simulink model "cdma_anti_jamming_system"  (R2020b)
settings: Solver=VariableStepAuto  StartTime=0.0  StopTime=0.004  RelTol=1e-3
undefined symbols (not defined in the file): fdesignblkfcn, gcbh
libraries: commutil2 x5, commfilt2 x1, commchan3 x1, commrandsrc3 x1, commseqgen3 x1
settings Model: Creator=joycelai  LastModifiedBy=joycelai

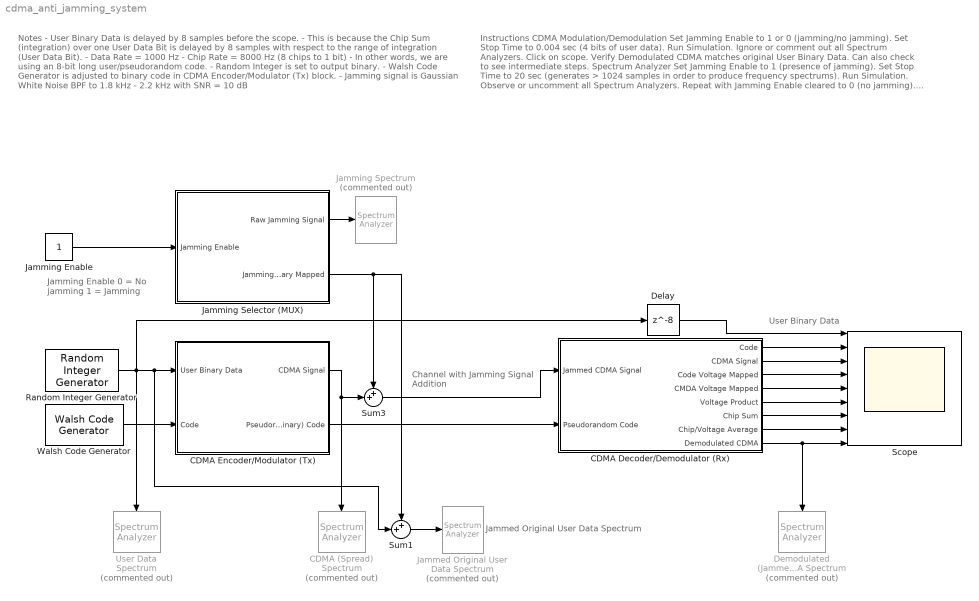
== system cdma_anti_jamming_system ==
  note: Jammed Original User Data Spectrum
  note: Jamming Enable
      | 0 = No jamming
      | 1 = Jamming
  note: Notes
      |
      | - User Binary Data is delayed by 8 samples before the scope.
      | - This is because the Chip Sum (integration) over one User Data Bit is delayed by 8 samples with respect to the range of integration (User Data Bit).
      |
      | - Data Rate = 1000 Hz
      | - Chip Rate = 8000 Hz (8 chips to 1 bit)
      | - In other words, we are using an 8-bit long user/pseudorandom code.
      | - Random Integer is set to output binary.
      | - Walsh Code Generator is adjusted to binary code in CDMA Encoder/Modulator (Tx) block.
      | - Jamming signal is Gaussian White Noise BPF to 1.8 kHz - 2.2 kHz with SNR = 10 dB
  note: Instructions
      |
      | CDMA Modulation/Demodulation
      |
      | Set Jamming Enable to 1 or 0 (jamming/no jamming).
      | Set Stop Time to 0.004 sec (4 bits of user data).
      | Run Simulation.
      | Ignore or comment out all Spectrum Analyzers.
      | Click on scope.
      | Verify Demodulated CDMA matches original User Binary Data.
      | Can also check to see intermediate steps.
      |
      | Spectrum Analyzer
      |
      | Set Jamming Enable to 1 (presence of jamming).
      | Set Stop Time to 20 sec (generates > 1024 samples in order to produce frequency spectrums).
      | Run Simulation.
      | Observe or uncomment all Spectrum Analyzers.
      | Repeat with Jamming Enable cleared to 0 (no jamming).
      | Verify that the Demodulated (Jammed) CDMA Spectrum mirrors the User Data Spectrum.
  note: User Binary Data
  note: Channel with Jamming Signal Addition
  CDMA (Spread) Spectrum : SpectrumAnalyzer  Commented=on
  CDMA Decoder/Demodulator (Rx) : Subsystem
  CDMA Encoder/Modulator (Tx) : Subsystem
  Delay : Delay  DelayLength=8  InitialCondition=0  SampleTime=1/(1000*8)
  Demodulated (Jammed) CDMA Spectrum : SpectrumAnalyzer  Commented=on
  Jammed Original User Data Spectrum : SpectrumAnalyzer  Commented=on
  Jamming Enable : Constant
  Jamming Selector (MUX) : Subsystem
  Jamming Spectrum : SpectrumAnalyzer  Commented=on
  Random Integer Generator : commrandsrc3/Random Integer Generator  SetSize=2  SeedSource=Auto  Seed=10  SampleTime=1/1000  SamplesPerFrame=1  OutputDataType=double  SimulateUsing=Interpreted execution
  Scope : Scope  NumInputPorts=9
  Sum1 : Sum  Inputs=++|
  Sum3 : Sum  Inputs=++|
  User Data Spectrum : SpectrumAnalyzer  Commented=on
  Walsh Code Generator : commseqgen3/Walsh Code Generator  Length=8  Index=5  SampleTime=1/(1000*8)  SamplesPerFrame=1  OutputDataType=double  SimulateUsing=Code generation
      settings: SourceProductBaseCode=CM
  wires:
  Walsh Code Generator/1 -> CDMA Encoder/Modulator (Tx)/2(Code)
  Sum3/1 -> CDMA Decoder/Demodulator (Rx)/1(Jammed CDMA Signal)
  CDMA Decoder/Demodulator (Rx)/8(Demodulated CDMA) -> Scope/9, Demodulated (Jammed) CDMA Spectrum/1
  Random Integer Generator/1 -> CDMA Encoder/Modulator (Tx)/1(User Binary Data), Sum1/2, Delay/1, User Data Spectrum/1
  Jamming Selector (MUX)/1(Raw Jamming Signal) -> Jamming Spectrum/1
  Jamming Selector (MUX)/2(Jamming Binary Mapped) -> Sum3/1, Sum1/1
  Jamming Enable/1 -> Jamming Selector (MUX)/1(Jamming Enable)
  CDMA Decoder/Demodulator (Rx)/7(Chip/Voltage Average) -> Scope/8
  CDMA Decoder/Demodulator (Rx)/6(Chip Sum) -> Scope/7
  CDMA Decoder/Demodulator (Rx)/5(Voltage Product) -> Scope/6
  CDMA Decoder/Demodulator (Rx)/4(CMDA Voltage Mapped) -> Scope/5
  CDMA Decoder/Demodulator (Rx)/3(Code Voltage Mapped) -> Scope/4
  CDMA Decoder/Demodulator (Rx)/2(CDMA Signal) -> Scope/3
  CDMA Decoder/Demodulator (Rx)/1(Code) -> Scope/2
  CDMA Encoder/Modulator (Tx)/2(Pseudorandom (Binary) Code) -> CDMA Decoder/Demodulator (Rx)/2(Pseudorandom Code)
  Delay/1 -> Scope/1
  Sum1/1 -> Jammed Original User Data Spectrum/1
  CDMA Encoder/Modulator (Tx)/1(CDMA Signal) -> Sum3/2, CDMA (Spread) Spectrum/1

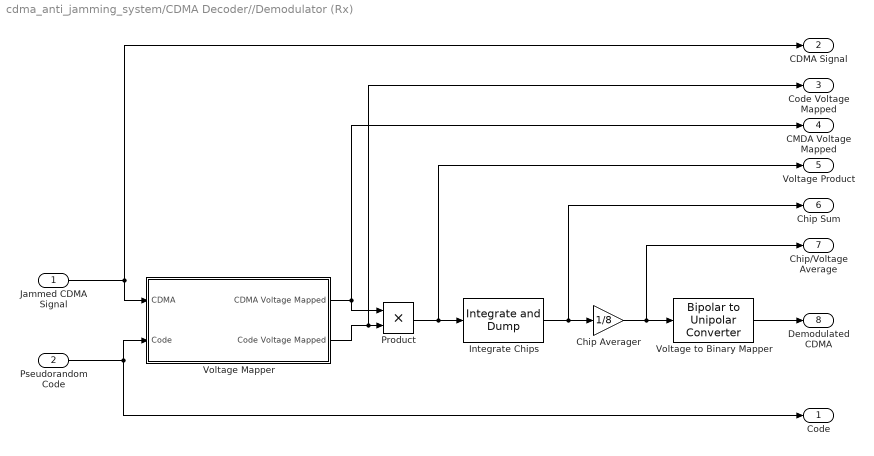
== system cdma_anti_jamming_system/CDMA Decoder//Demodulator (Rx) ==
  Jammed CDMA Signal : Inport
  Pseudorandom Code : Inport  Port=2
  Chip Averager : Gain  Gain=1/8
  Integrate Chips : commfilt2/Integrate and Dump  obssamples=8  offsetsamples=0  nodump=off  roundingMode=Floor  overflowMode=off  outputDataTypeStr=Inherit: Same as accumulator  outputLastDataTypeStr=Inherit: Same as accumulator
  Product : Product
  Voltage Mapper : Subsystem
  Voltage to Binary Mapper : commutil2/Bipolar to Unipolar Converter  M=2  polarity=Negative  dataType=Inherit via internal rule
      settings: SourceProductBaseCode=CM
  Code : Outport
  CDMA Signal : Outport  Port=2
  Code Voltage Mapped : Outport  Port=3
  CMDA Voltage Mapped : Outport  Port=4
  Voltage Product : Outport  Port=5
  Chip Sum : Outport  Port=6
  Chip/Voltage Average : Outport  Port=7
  Demodulated CDMA : Outport  Port=8
  wires:
  Chip Averager/1 -> Chip/Voltage Average/1, Voltage to Binary Mapper/1
  Voltage to Binary Mapper/1 -> Demodulated CDMA/1
  Voltage Mapper/2(Code Voltage Mapped) -> Code Voltage Mapped/1, Product/2
  Integrate Chips/1 -> Chip Sum/1, Chip Averager/1
  Voltage Mapper/1(CDMA Voltage Mapped) -> Product/1, CMDA Voltage Mapped/1
  Product/1 -> Voltage Product/1, Integrate Chips/1
  Jammed CDMA Signal/1 -> CDMA Signal/1, Voltage Mapper/1(CDMA)
  Pseudorandom Code/1 -> Code/1, Voltage Mapper/2(Code)

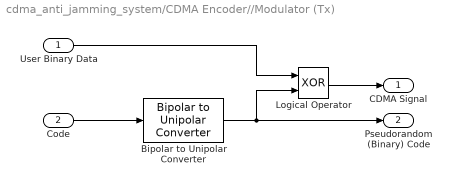
== system cdma_anti_jamming_system/CDMA Encoder//Modulator (Tx) ==
  User Binary Data : Inport
  Code : Inport  Port=2
  Bipolar to Unipolar Converter : commutil2/Bipolar to Unipolar Converter  M=2  polarity=Positive  dataType=Inherit via internal rule
      settings: SourceProductBaseCode=CM
  Logical Operator : Logic  Operator=XOR  AllPortsSameDT=off  OutDataTypeStr=boolean
  CDMA Signal : Outport
  Pseudorandom (Binary) Code : Outport  Port=2
  wires:
  User Binary Data/1 -> Logical Operator/1
  Code/1 -> Bipolar to Unipolar Converter/1
  Bipolar to Unipolar Converter/1 -> Pseudorandom (Binary) Code/1, Logical Operator/2
  Logical Operator/1 -> CDMA Signal/1

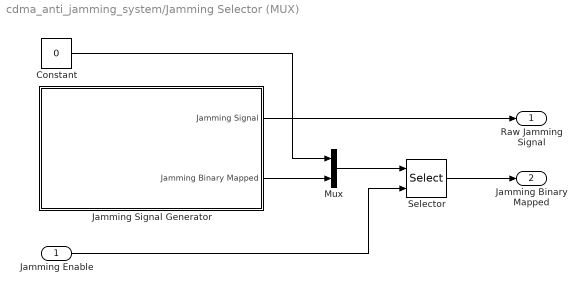
== system cdma_anti_jamming_system/Jamming Selector (MUX) ==
  Jamming Enable : Inport
  Constant : Constant  Value=0  SampleTime=1/1000
  Jamming Signal Generator : Subsystem
  Mux : Mux  Inputs=2
  Selector : Selector  IndexMode=Zero-based  InputPortWidth=2  IndexOptions=Index vector (port)  Indices=0  OutputSizes=1
  Raw Jamming Signal : Outport
  Jamming Binary Mapped : Outport  Port=2
  wires:
  Jamming Signal Generator/2(Jamming Binary Mapped) -> Mux/2
  Constant/1 -> Mux/1
  Selector/1 -> Jamming Binary Mapped/1
  Jamming Signal Generator/1(Jamming Signal) -> Raw Jamming Signal/1
  Mux/1 -> Selector/1
  Jamming Enable/1 -> Selector/2

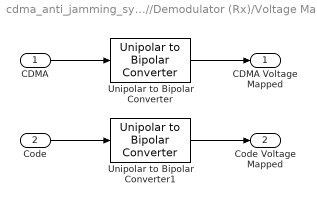
== system cdma_anti_jamming_system/CDMA Decoder//Demodulator (Rx)/Voltage Mapper ==
  CDMA : Inport
  Code : Inport  Port=2
  Unipolar to Bipolar Converter : commutil2/Unipolar to Bipolar Converter  M=2  polarity=Negative  dataType=Inherit via internal rule
  Unipolar to Bipolar Converter1 : commutil2/Unipolar to Bipolar Converter  M=2  polarity=Negative  dataType=Inherit via internal rule
  CDMA Voltage Mapped : Outport
  Code Voltage Mapped : Outport  Port=2
  wires:
  CDMA/1 -> Unipolar to Bipolar Converter/1
  Code/1 -> Unipolar to Bipolar Converter1/1
  Unipolar to Bipolar Converter/1 -> CDMA Voltage Mapped/1
  Unipolar to Bipolar Converter1/1 -> Code Voltage Mapped/1

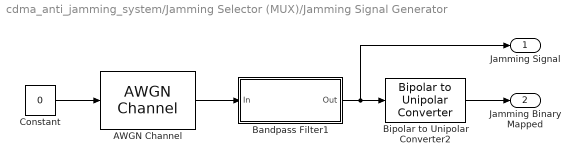
== system cdma_anti_jamming_system/Jamming Selector (MUX)/Jamming Signal Generator ==
  AWGN Channel : commchan3/AWGN Channel  InputProcessing=Columns as channels (frame based)  seed=67  noiseMode="Signal to noise ratio  (SNR)"  EbNodB=10  EsNodB=10  SNRdB=10  bitsPerSym=1  Ps=1  Tsym=1  variance=1
  Bandpass Filter1 : Subsystem  DialogController=fdesignblkfcn  InitFcn=fdesignblkfcn(gcbh, {'InitFcn'});  mask(Bandpass Filter){}
      mask help: Design a bandpass filter
      settings: CopyFcn=fdesignblkfcn(gcbh, {'CopyFcn'});
      mask Help: helpview(mapfilelocation('dsp'), 'dspbandpassfilter');
      mask Display: disp('Bandpass');
  Bipolar to Unipolar Converter2 : commutil2/Bipolar to Unipolar Converter  M=2  polarity=Positive  dataType=Inherit via internal rule
      settings: SourceProductBaseCode=CM
  Constant : Constant  Value=0  SampleTime=1/1000
  Jamming Signal : Outport
  Jamming Binary Mapped : Outport  Port=2
  wires:
  Constant/1 -> AWGN Channel/1
  AWGN Channel/1 -> Bandpass Filter1/1(In)
  Bipolar to Unipolar Converter2/1 -> Jamming Binary Mapped/1
  Bandpass Filter1/1(Out) -> Jamming Signal/1, Bipolar to Unipolar Converter2/1

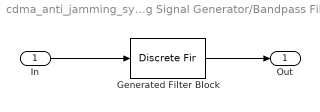
== system cdma_anti_jamming_system/Jamming Selector (MUX)/Jamming Signal Generator/Bandpass Filter1 ==
  In : Inport
  Generated Filter Block : DiscreteFir  Tag=BlockMethodSubSystem  Coefficients=[-0.0008992291487744296 0.0016414518747943749 0.0031352071842225397 -0.0040707550828814922 -0.0063731852227904111 0.0074874286806090491 0.0098354319566295711 -0.010189316513446216 -0.011302794465874122 0.0096929185841818435 0.0079428653987464216 -0.0031368247881221642 0.0028299878877943137 -0.011508674243001471 -0.022080136219461581 0.034245325424507672 0.048356661648905473 -0.062355369169884239 -0.077503478162593897 0.090687768153125653 0.10353171105844157 -0.11297860084229834 -0.12035866024978455 0.12379360801539134 0.12379360801539134 -0.12035866024978455 -0.11297860084229834 0.10353171105844157 0.090687768153125653 -0.077503478162593897 -0.062355369169884239 0.048356661648905473 0.034245325424507672 -0.022080136219461581 -0.011508674243001471 0.0028299878877943137 -0.0031368247881221642 0.0079428653987464216 0.0096929185841818435 -0.011302794465874122 -0.010189316513446216 0.0098354319566295711 0.0074874286806090491 -0.0063731852227904111 -0.0040707550828814922 0.0031352071842225397 0.0016414518747943749 -0.0008992291487744296]  InputProcessing=Columns as channels (frame based)
  Out : Outport  VectorParamsAs1DForOutWhenUnconnected=off
  wires:
  In/1 -> Generated Filter Block/1
  Generated Filter Block/1 -> Out/1
